simulink model "PV_Array_Application_R"  (Simulink 7.5)
settings: Solver=ode1  StartTime=0.0  StopTime=10.0  FixedStep=0.01  RelTol=1e-3
libraries: simulink x8, powerlib x4
settings Model: Creator=Leo216  LastModifiedBy=Leo216

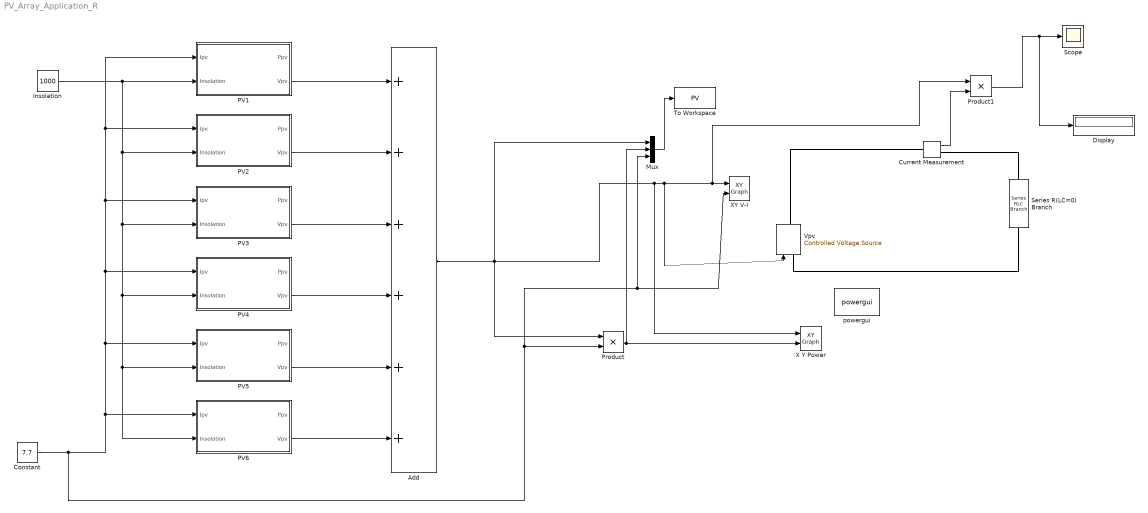
== system PV_Array_Application_R ==
  Add : Sum  Inputs=++++++  OutDataType=fixdt(1, 16)  OutScaling=2^-10
  Constant : Constant  Value=7.7  OutDataType=fixdt(1, 16)  OutScaling=2^0
  Current Measurement : powerlib/Measurements/Current Measurement  DialogController=POWERSYS.PowerSysDialog  SystemSampleTime=-1  PhasorSimulation=off  OutputType=Complex  PSBequivalent=0
  Display : Display
  Insolation : Constant  Value=1000  OutDataType=fixdt(1, 16)  OutScaling=2^0  SampleTime=-1
  Mux : Mux  Inputs=3
  PV1 : Subsystem  mask{Isc=8.4, Voc=39.6/63, Ir=7.7, Vr=31.9/63, Diode=on}
      mask prompts: Isc "Short-circuit current"; Voc "Open-Circuit Voltage"; Ir "Current at Pmax"; Vr "Voltage at Pmax"; Diode "By-pass diode"
      mask init:
      | Ns=round(Voc/0.61);
      | Vt=26e-3
      | G= Isc/1000;
      | Vmpc=Vr/Ns;
      | Vocc=Voc/Ns;
      | Rmpp=Vmpc/Ir;
      | 
      | Rp=100*Vocc/Isc;
      | Vdm=Vocc;
      | 
      | for i=1:10
      |     
      |    Idm=Isc-Ir-Vdm/Rp;
      |    Io=(Isc-Vocc/Rp)/(exp(Vocc/Vt)-1);
      |    Vdm=Vt*log(Idm/Io+1);
      |    Rs=(Vdm-Vmpc)/Ir;
      |    Rd=(Rmpp-Rs)*Rp/(Rp-Rmpp+Rs);
      |    Idm=Vt/Rd;
      |    Rp=Vdm/(Isc-Ir-Idm);
      |    
      | end
      mask Display: image(imread('pv.jpg'))
  PV2 : Subsystem  mask{Isc=8.4, Voc=39.6/63, Ir=7.7, Vr=31.9/63, Diode=on}
      mask prompts: Isc "Short-circuit current"; Voc "Open-Circuit Voltage"; Ir "Current at Pmax"; Vr "Voltage at Pmax"; Diode "By-pass diode"
      mask init: same as PV_Array_Application_R/PV1
      mask Display: image(imread('pv.jpg'))
  PV3 : Subsystem  mask{Isc=8.4, Voc=39.6/63, Ir=7.7, Vr=31.9/63, Diode=on}
      mask prompts: Isc "Short-circuit current"; Voc "Open-Circuit Voltage"; Ir "Current at Pmax"; Vr "Voltage at Pmax"; Diode "By-pass diode"
      mask init: same as PV_Array_Application_R/PV1
      mask Display: image(imread('pv.jpg'))
  PV4 : Subsystem  mask{Isc=8.4, Voc=39.6/63, Ir=7.7, Vr=31.9/63, Diode=on}
      mask prompts: Isc "Short-circuit current"; Voc "Open-Circuit Voltage"; Ir "Current at Pmax"; Vr "Voltage at Pmax"; Diode "By-pass diode"
      mask init: same as PV_Array_Application_R/PV1
      mask Display: image(imread('pv.jpg'))
  PV5 : Subsystem  mask{Isc=8.4, Voc=39.6/63, Ir=7.7, Vr=31.9/63, Diode=on}
      mask prompts: Isc "Short-circuit current"; Voc "Open-Circuit Voltage"; Ir "Current at Pmax"; Vr "Voltage at Pmax"; Diode "By-pass diode"
      mask init: same as PV_Array_Application_R/PV1
      mask Display: image(imread('pv.jpg'))
  PV6 : Subsystem  mask{Isc=8.4, Voc=39.6/63, Ir=7.7, Vr=31.9/63, Diode=on}
      mask prompts: Isc "Short-circuit current"; Voc "Open-Circuit Voltage"; Ir "Current at Pmax"; Vr "Voltage at Pmax"; Diode "By-pass diode"
      mask init: same as PV_Array_Application_R/PV1
      mask Display: image(imread('pv.jpg'))
  Product : Product  OutDataType=fixdt(1, 16)  OutScaling=2^0  RndMeth=Zero
  Product1 : Product  OutDataType=fixdt(1, 16)  OutScaling=2^0  RndMeth=Zero
  Scope : Scope
      settings: TimeRange=50
  Series R(LC=0) Branch : powerlib/Elements/Series RLC Branch  DialogController=POWERSYS.PowerSysDialog  PhysicalDomain=powersysdomain  SubClassName=unknown  LeftPortType=p1  RightPortType=p1  LConnTagsString=__new0  RConnTagsString=__new0  BranchType=R  Resistance=0.39  Inductance=1e-3  SetiL0=off  InitialCurrent=0  Capacitance=1e-6  Setx0=off  InitialVoltage=0  Measurements=None
  To Workspace : ToWorkspace  VariableName=PV  SampleTime=-1  SaveFormat=Structure
  Vpv : powerlib/Electrical Sources/Controlled Voltage Source  DialogController=POWERSYS.PowerSysDialog  SystemSampleTime=-1  Initialize=on  Source_Type=AC  Amplitude=0  Phase=0  Frequency=0  Measurements=None
  X Y Power : simulink/Sinks/XY Graph  SystemSampleTime=-1  xmin=0  xmax=10  ymin=0  ymax=10  st=-1
  XY V-I : simulink/Sinks/XY Graph  SystemSampleTime=-1  xmin=0  xmax=10  ymin=0  ymax=10  st=-1
  powergui : powerlib/powergui  Priority=1  SystemSampleTime=-1  SimulationMode=Continuous  SampleTime=50e-6  frequency=60  SPID=off  DisableSnubberDevices=off  DisableRonSwitches=off  DisableVfSwitches=off  SwTol=0  Interpol=off  frequencyindice=0  echomessages=off  HookPort=off  DisplayEquations=off  FunctionMessages=off  EnableUseOfTLC=off  x0status=blocks  RestoreLinks=warning  ResistiveCurrentMeasurement=off  Ylog=off  Xlog=on  ShowGrid=off  save=off  variable=ZData  ZoomFFT=off  StartTime=0.0  cycles=1  DisplayStyle=1  FreqAxis=off  MaxFrequency=1000  frequencyindicesteady=1  display=off  methode=off
  wires:
  PV1/2(Vpv) -> Add/1
  PV2/2(Vpv) -> Add/2
  PV3/2(Vpv) -> Add/3
  PV4/2(Vpv) -> Add/4
  PV5/2(Vpv) -> Add/5
  PV6/2(Vpv) -> Add/6
  Insolation/1 -> PV1/2(Insolation), PV5/2(Insolation), PV6/2(Insolation), PV4/2(Insolation), PV3/2(Insolation), PV2/2(Insolation)
  Constant/1 -> PV1/1(Ipv), PV2/1(Ipv), PV3/1(Ipv), PV4/1(Ipv), PV5/1(Ipv), PV6/1(Ipv), Product/2, XY V-I/2, Mux/3
  Product/1 -> X Y Power/2, Mux/2
  Mux/1 -> To Workspace/1
  Add/1 -> Mux/1, X Y Power/1, Vpv/1, XY V-I/1, Product1/1, Product/1
  Current Measurement/1 -> Product1/2
  Product1/1 -> Scope/1, Display/1
  connections:
  Vpv/LConn1 -- Series R(LC=0) Branch/RConn1
  Vpv/RConn1 -- Current Measurement/LConn1
  Current Measurement/RConn1 -- Series R(LC=0) Branch/LConn1

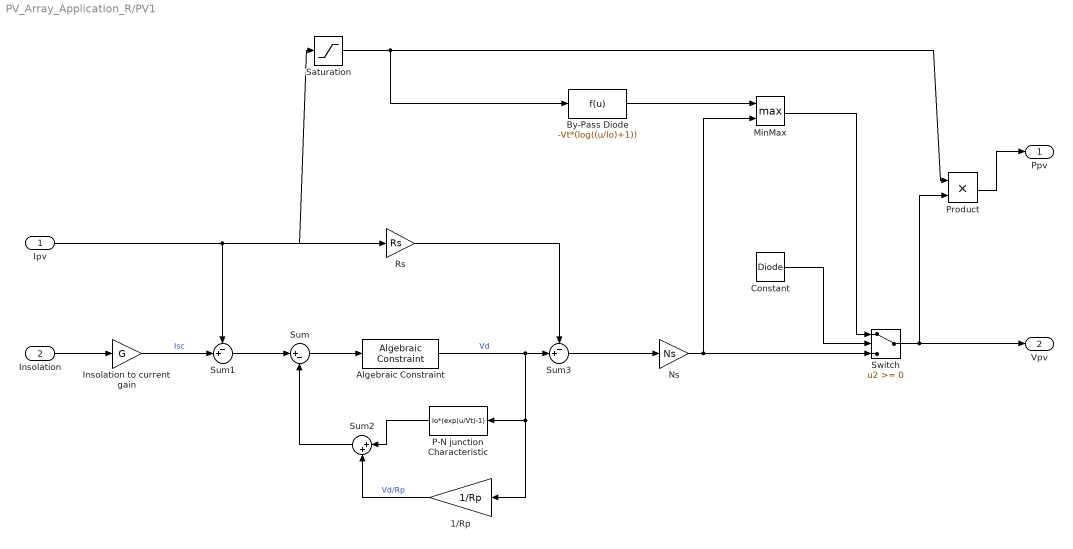
== system PV_Array_Application_R/PV1 ==
  Ipv : Inport  OutDataType=fixdt(1, 16)  OutScaling=2^0
  Insolation : Inport  Port=2  OutDataType=fixdt(1, 16)  OutScaling=2^0
  1/Rp : Gain  Gain=1/Rp  ParameterDataType=fixdt(1, 16)  ParameterScaling=2^0  OutDataType=fixdt(1, 16)  OutScaling=2^0
  Algebraic Constraint : simulink/Math Operations/Algebraic Constraint  SystemSampleTime=-1  z0=0.5
  By-Pass Diode : Fcn  Expr=-Vt*(log((u/Io)+1))
  Constant : Constant  Value=Diode  OutDataType=fixdt(1, 16)  OutScaling=2^0  SampleTime=-1
  Insolation to current gain : Gain  Gain=G  ParameterDataType=fixdt(1, 16)  ParameterScaling=2^0  OutDataType=fixdt(1, 16)  OutScaling=2^0
  MinMax : MinMax  Function=max  Inputs=2  OutDataType=fixdt(1, 16)  OutScaling=2^0
  Ns : Gain  Gain=Ns  ParameterDataType=fixdt(1, 16)  ParameterScaling=2^0  OutDataType=fixdt(1, 16)  OutScaling=2^0
  P-N junction Characteristic : Fcn  Expr=Io*(exp(u/Vt)-1)
  Product : Product  OutDataType=fixdt(1, 16)  OutScaling=2^0  RndMeth=Zero
  Rs : Gain  Gain=Rs  ParameterDataType=fixdt(1, 16)  ParameterScaling=2^0  OutDataType=fixdt(1, 16)  OutScaling=2^0
  Saturation : Saturate  OutDataType=fixdt(1, 16)  OutScaling=2^0
  Sum : Sum  Inputs=|+-  OutDataType=fixdt(1, 16)  OutScaling=2^0
  Sum1 : Sum  Inputs=-+|  OutDataType=fixdt(1, 16)  OutScaling=2^0
  Sum2 : Sum  Inputs=|++  OutDataType=fixdt(1, 16)  OutScaling=2^0
  Sum3 : Sum  Inputs=-+|  OutDataType=fixdt(1, 16)  OutScaling=2^0
  Switch : Switch  OutDataType=fixdt(1, 16)  OutScaling=2^0
  Ppv : Outport  OutDataType=fixdt(1, 16)  OutScaling=2^0
  Vpv : Outport  Port=2  OutDataType=fixdt(1, 16)  OutScaling=2^0
  wires:
  Insolation/1 -> Insolation to current gain/1
  Product/1 -> Ppv/1
  By-Pass Diode/1 -> MinMax/1
  P-N junction Characteristic/1 -> Sum2/1
  Saturation/1 -> Product/1, By-Pass Diode/1
  Switch/1 -> Product/2, Vpv/1
  MinMax/1 -> Switch/1
  Constant/1 -> Switch/2
  Ns/1 -> Switch/3, MinMax/2
  Sum3/1 -> Ns/1
  Rs/1 -> Sum3/1
  Algebraic Constraint/1 -> Sum3/2, 1/Rp/1, P-N junction Characteristic/1  "Vd"
  1/Rp/1 -> Sum2/2  "Vd/Rp"
  Sum2/1 -> Sum/2
  Sum/1 -> Algebraic Constraint/1
  Sum1/1 -> Sum/1
  Insolation to current gain/1 -> Sum1/2  "Isc"
  Ipv/1 -> Sum1/1, Rs/1, Saturation/1

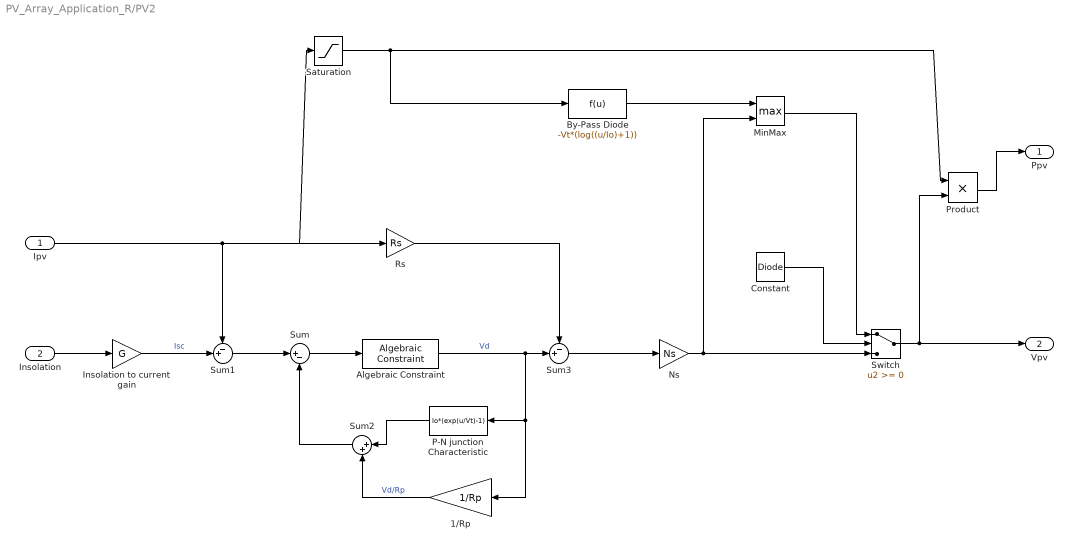
== system PV_Array_Application_R/PV2 ==
  Ipv : Inport  OutDataType=fixdt(1, 16)  OutScaling=2^0
  Insolation : Inport  Port=2  OutDataType=fixdt(1, 16)  OutScaling=2^0
  1/Rp : Gain  Gain=1/Rp  ParameterDataType=fixdt(1, 16)  ParameterScaling=2^0  OutDataType=fixdt(1, 16)  OutScaling=2^0
  Algebraic Constraint : simulink/Math Operations/Algebraic Constraint  SystemSampleTime=-1  z0=0
  By-Pass Diode : Fcn  Expr=-Vt*(log((u/Io)+1))
  Constant : Constant  Value=Diode  OutDataType=fixdt(1, 16)  OutScaling=2^0  SampleTime=-1
  Insolation to current gain : Gain  Gain=G  ParameterDataType=fixdt(1, 16)  ParameterScaling=2^0  OutDataType=fixdt(1, 16)  OutScaling=2^0
  MinMax : MinMax  Function=max  Inputs=2  OutDataType=fixdt(1, 16)  OutScaling=2^0
  Ns : Gain  Gain=Ns  ParameterDataType=fixdt(1, 16)  ParameterScaling=2^0  OutDataType=fixdt(1, 16)  OutScaling=2^0
  P-N junction Characteristic : Fcn  Expr=Io*(exp(u/Vt)-1)
  Product : Product  OutDataType=fixdt(1, 16)  OutScaling=2^0  RndMeth=Zero
  Rs : Gain  Gain=Rs  ParameterDataType=fixdt(1, 16)  ParameterScaling=2^0  OutDataType=fixdt(1, 16)  OutScaling=2^0
  Saturation : Saturate  OutDataType=fixdt(1, 16)  OutScaling=2^0
  Sum : Sum  Inputs=|+-  OutDataType=fixdt(1, 16)  OutScaling=2^0
  Sum1 : Sum  Inputs=-+|  OutDataType=fixdt(1, 16)  OutScaling=2^0
  Sum2 : Sum  Inputs=|++  OutDataType=fixdt(1, 16)  OutScaling=2^0
  Sum3 : Sum  Inputs=-+|  OutDataType=fixdt(1, 16)  OutScaling=2^0
  Switch : Switch  OutDataType=fixdt(1, 16)  OutScaling=2^0
  Ppv : Outport  OutDataType=fixdt(1, 16)  OutScaling=2^0
  Vpv : Outport  Port=2  OutDataType=fixdt(1, 16)  OutScaling=2^0
  wires:
  Insolation/1 -> Insolation to current gain/1
  Product/1 -> Ppv/1
  By-Pass Diode/1 -> MinMax/1
  P-N junction Characteristic/1 -> Sum2/1
  Saturation/1 -> Product/1, By-Pass Diode/1
  Switch/1 -> Product/2, Vpv/1
  MinMax/1 -> Switch/1
  Constant/1 -> Switch/2
  Ns/1 -> Switch/3, MinMax/2
  Sum3/1 -> Ns/1
  Rs/1 -> Sum3/1
  Algebraic Constraint/1 -> Sum3/2, 1/Rp/1, P-N junction Characteristic/1  "Vd"
  1/Rp/1 -> Sum2/2  "Vd/Rp"
  Sum2/1 -> Sum/2
  Sum/1 -> Algebraic Constraint/1
  Sum1/1 -> Sum/1
  Insolation to current gain/1 -> Sum1/2  "Isc"
  Ipv/1 -> Sum1/1, Rs/1, Saturation/1

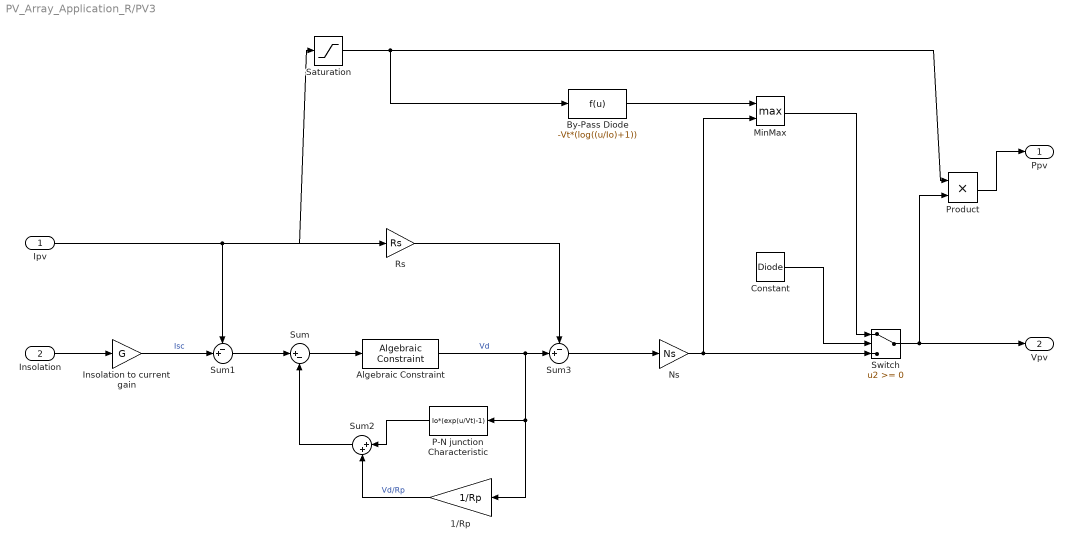
== system PV_Array_Application_R/PV3 ==
  Ipv : Inport  OutDataType=fixdt(1, 16)  OutScaling=2^0
  Insolation : Inport  Port=2  OutDataType=fixdt(1, 16)  OutScaling=2^0
  1/Rp : Gain  Gain=1/Rp  ParameterDataType=fixdt(1, 16)  ParameterScaling=2^0  OutDataType=fixdt(1, 16)  OutScaling=2^0
  Algebraic Constraint : simulink/Math Operations/Algebraic Constraint  SystemSampleTime=-1  z0=0
  By-Pass Diode : Fcn  Expr=-Vt*(log((u/Io)+1))
  Constant : Constant  Value=Diode  OutDataType=fixdt(1, 16)  OutScaling=2^0  SampleTime=-1
  Insolation to current gain : Gain  Gain=G  ParameterDataType=fixdt(1, 16)  ParameterScaling=2^0  OutDataType=fixdt(1, 16)  OutScaling=2^0
  MinMax : MinMax  Function=max  Inputs=2  OutDataType=fixdt(1, 16)  OutScaling=2^0
  Ns : Gain  Gain=Ns  ParameterDataType=fixdt(1, 16)  ParameterScaling=2^0  OutDataType=fixdt(1, 16)  OutScaling=2^0
  P-N junction Characteristic : Fcn  Expr=Io*(exp(u/Vt)-1)
  Product : Product  OutDataType=fixdt(1, 16)  OutScaling=2^0  RndMeth=Zero
  Rs : Gain  Gain=Rs  ParameterDataType=fixdt(1, 16)  ParameterScaling=2^0  OutDataType=fixdt(1, 16)  OutScaling=2^0
  Saturation : Saturate  OutDataType=fixdt(1, 16)  OutScaling=2^0
  Sum : Sum  Inputs=|+-  OutDataType=fixdt(1, 16)  OutScaling=2^0
  Sum1 : Sum  Inputs=-+|  OutDataType=fixdt(1, 16)  OutScaling=2^0
  Sum2 : Sum  Inputs=|++  OutDataType=fixdt(1, 16)  OutScaling=2^0
  Sum3 : Sum  Inputs=-+|  OutDataType=fixdt(1, 16)  OutScaling=2^0
  Switch : Switch  OutDataType=fixdt(1, 16)  OutScaling=2^0
  Ppv : Outport  OutDataType=fixdt(1, 16)  OutScaling=2^0
  Vpv : Outport  Port=2  OutDataType=fixdt(1, 16)  OutScaling=2^0
  wires:
  Insolation/1 -> Insolation to current gain/1
  Product/1 -> Ppv/1
  By-Pass Diode/1 -> MinMax/1
  P-N junction Characteristic/1 -> Sum2/1
  Saturation/1 -> Product/1, By-Pass Diode/1
  Switch/1 -> Product/2, Vpv/1
  MinMax/1 -> Switch/1
  Constant/1 -> Switch/2
  Ns/1 -> Switch/3, MinMax/2
  Sum3/1 -> Ns/1
  Rs/1 -> Sum3/1
  Algebraic Constraint/1 -> Sum3/2, 1/Rp/1, P-N junction Characteristic/1  "Vd"
  1/Rp/1 -> Sum2/2  "Vd/Rp"
  Sum2/1 -> Sum/2
  Sum/1 -> Algebraic Constraint/1
  Sum1/1 -> Sum/1
  Insolation to current gain/1 -> Sum1/2  "Isc"
  Ipv/1 -> Sum1/1, Rs/1, Saturation/1

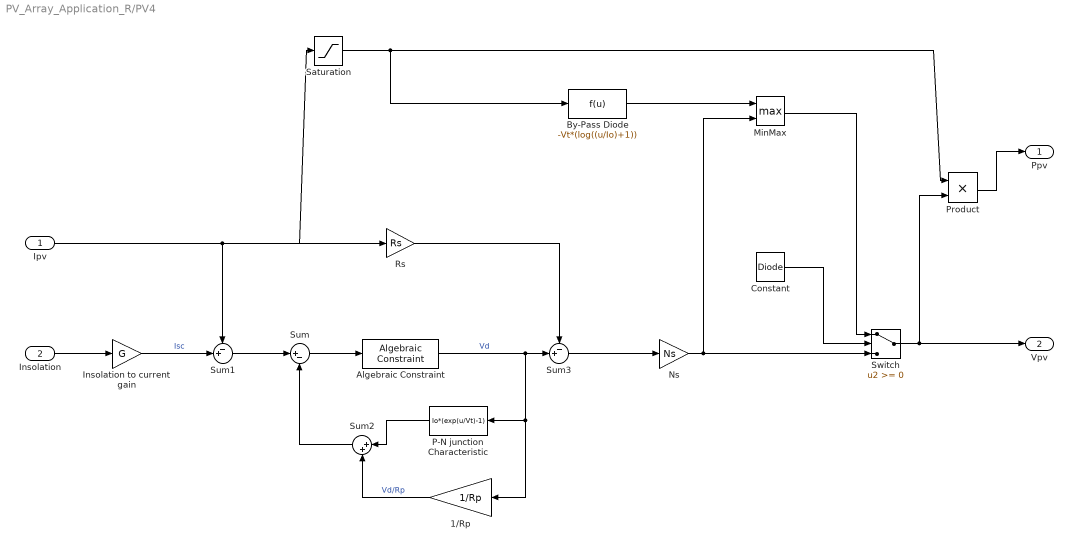
== system PV_Array_Application_R/PV4 ==
  Ipv : Inport  OutDataType=fixdt(1, 16)  OutScaling=2^0
  Insolation : Inport  Port=2  OutDataType=fixdt(1, 16)  OutScaling=2^0
  1/Rp : Gain  Gain=1/Rp  ParameterDataType=fixdt(1, 16)  ParameterScaling=2^0  OutDataType=fixdt(1, 16)  OutScaling=2^0
  Algebraic Constraint : simulink/Math Operations/Algebraic Constraint  SystemSampleTime=-1  z0=0
  By-Pass Diode : Fcn  Expr=-Vt*(log((u/Io)+1))
  Constant : Constant  Value=Diode  OutDataType=fixdt(1, 16)  OutScaling=2^0
  Insolation to current gain : Gain  Gain=G  ParameterDataType=fixdt(1, 16)  ParameterScaling=2^0  OutDataType=fixdt(1, 16)  OutScaling=2^0
  MinMax : MinMax  Function=max  Inputs=2  OutDataType=fixdt(1, 16)  OutScaling=2^0
  Ns : Gain  Gain=Ns  ParameterDataType=fixdt(1, 16)  ParameterScaling=2^0  OutDataType=fixdt(1, 16)  OutScaling=2^0
  P-N junction Characteristic : Fcn  Expr=Io*(exp(u/Vt)-1)
  Product : Product  OutDataType=fixdt(1, 16)  OutScaling=2^0  RndMeth=Zero
  Rs : Gain  Gain=Rs  ParameterDataType=fixdt(1, 16)  ParameterScaling=2^0  OutDataType=fixdt(1, 16)  OutScaling=2^0
  Saturation : Saturate  OutDataType=fixdt(1, 16)  OutScaling=2^0
  Sum : Sum  Inputs=|+-  OutDataType=fixdt(1, 16)  OutScaling=2^0
  Sum1 : Sum  Inputs=-+|  OutDataType=fixdt(1, 16)  OutScaling=2^0
  Sum2 : Sum  Inputs=|++  OutDataType=fixdt(1, 16)  OutScaling=2^0
  Sum3 : Sum  Inputs=-+|  OutDataType=fixdt(1, 16)  OutScaling=2^0
  Switch : Switch  OutDataType=fixdt(1, 16)  OutScaling=2^0
  Ppv : Outport  OutDataType=fixdt(1, 16)  OutScaling=2^0
  Vpv : Outport  Port=2  OutDataType=fixdt(1, 16)  OutScaling=2^0
  wires:
  Insolation/1 -> Insolation to current gain/1
  Product/1 -> Ppv/1
  By-Pass Diode/1 -> MinMax/1
  P-N junction Characteristic/1 -> Sum2/1
  Saturation/1 -> Product/1, By-Pass Diode/1
  Switch/1 -> Product/2, Vpv/1
  MinMax/1 -> Switch/1
  Constant/1 -> Switch/2
  Ns/1 -> Switch/3, MinMax/2
  Sum3/1 -> Ns/1
  Rs/1 -> Sum3/1
  Algebraic Constraint/1 -> Sum3/2, 1/Rp/1, P-N junction Characteristic/1  "Vd"
  1/Rp/1 -> Sum2/2  "Vd/Rp"
  Sum2/1 -> Sum/2
  Sum/1 -> Algebraic Constraint/1
  Sum1/1 -> Sum/1
  Insolation to current gain/1 -> Sum1/2  "Isc"
  Ipv/1 -> Sum1/1, Rs/1, Saturation/1

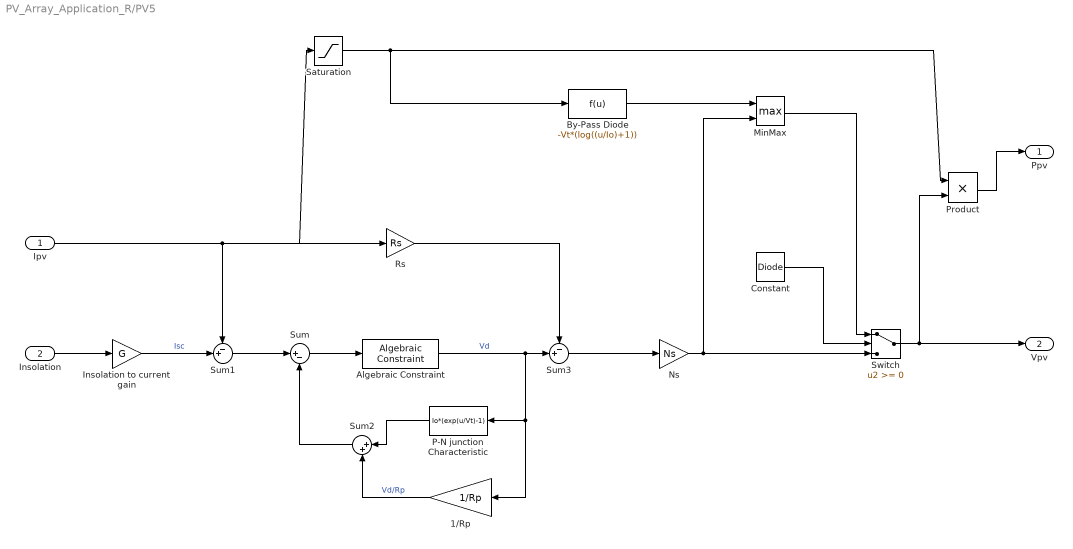
== system PV_Array_Application_R/PV5 ==
  Ipv : Inport  OutDataType=fixdt(1, 16)  OutScaling=2^0
  Insolation : Inport  Port=2  OutDataType=fixdt(1, 16)  OutScaling=2^0
  1/Rp : Gain  Gain=1/Rp  ParameterDataType=fixdt(1, 16)  ParameterScaling=2^0  OutDataType=fixdt(1, 16)  OutScaling=2^0
  Algebraic Constraint : simulink/Math Operations/Algebraic Constraint  SystemSampleTime=-1  z0=0
  By-Pass Diode : Fcn  Expr=-Vt*(log((u/Io)+1))
  Constant : Constant  Value=Diode  OutDataType=fixdt(1, 16)  OutScaling=2^0
  Insolation to current gain : Gain  Gain=G  ParameterDataType=fixdt(1, 16)  ParameterScaling=2^0  OutDataType=fixdt(1, 16)  OutScaling=2^0
  MinMax : MinMax  Function=max  Inputs=2  OutDataType=fixdt(1, 16)  OutScaling=2^0
  Ns : Gain  Gain=Ns  ParameterDataType=fixdt(1, 16)  ParameterScaling=2^0  OutDataType=fixdt(1, 16)  OutScaling=2^0
  P-N junction Characteristic : Fcn  Expr=Io*(exp(u/Vt)-1)
  Product : Product  OutDataType=fixdt(1, 16)  OutScaling=2^0  RndMeth=Zero
  Rs : Gain  Gain=Rs  ParameterDataType=fixdt(1, 16)  ParameterScaling=2^0  OutDataType=fixdt(1, 16)  OutScaling=2^0
  Saturation : Saturate  OutDataType=fixdt(1, 16)  OutScaling=2^0
  Sum : Sum  Inputs=|+-  OutDataType=fixdt(1, 16)  OutScaling=2^0
  Sum1 : Sum  Inputs=-+|  OutDataType=fixdt(1, 16)  OutScaling=2^0
  Sum2 : Sum  Inputs=|++  OutDataType=fixdt(1, 16)  OutScaling=2^0
  Sum3 : Sum  Inputs=-+|  OutDataType=fixdt(1, 16)  OutScaling=2^0
  Switch : Switch  OutDataType=fixdt(1, 16)  OutScaling=2^0
  Ppv : Outport  OutDataType=fixdt(1, 16)  OutScaling=2^0
  Vpv : Outport  Port=2  OutDataType=fixdt(1, 16)  OutScaling=2^0
  wires:
  Insolation/1 -> Insolation to current gain/1
  Product/1 -> Ppv/1
  By-Pass Diode/1 -> MinMax/1
  P-N junction Characteristic/1 -> Sum2/1
  Saturation/1 -> Product/1, By-Pass Diode/1
  Switch/1 -> Product/2, Vpv/1
  MinMax/1 -> Switch/1
  Constant/1 -> Switch/2
  Ns/1 -> Switch/3, MinMax/2
  Sum3/1 -> Ns/1
  Rs/1 -> Sum3/1
  Algebraic Constraint/1 -> Sum3/2, 1/Rp/1, P-N junction Characteristic/1  "Vd"
  1/Rp/1 -> Sum2/2  "Vd/Rp"
  Sum2/1 -> Sum/2
  Sum/1 -> Algebraic Constraint/1
  Sum1/1 -> Sum/1
  Insolation to current gain/1 -> Sum1/2  "Isc"
  Ipv/1 -> Sum1/1, Rs/1, Saturation/1

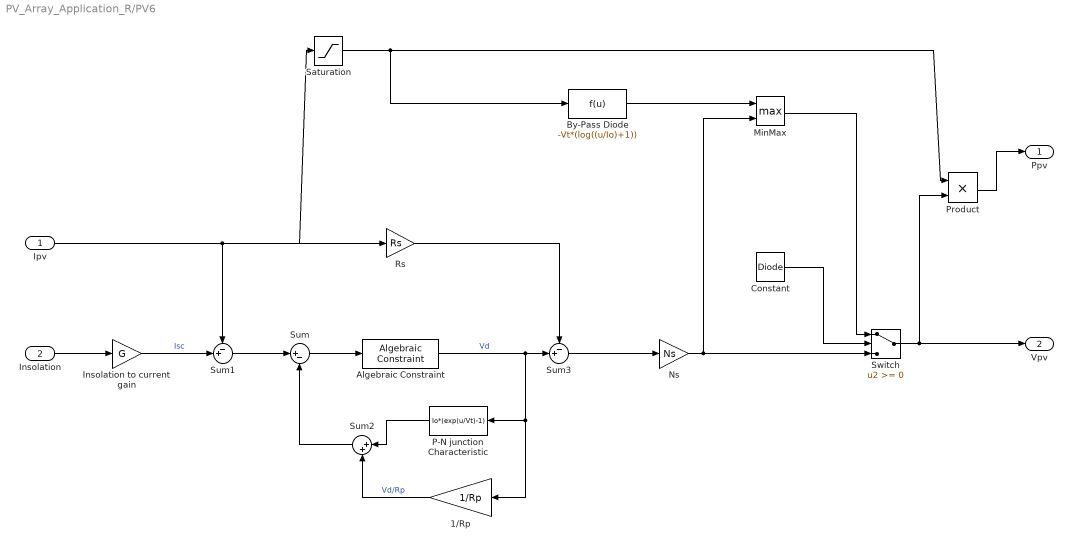
== system PV_Array_Application_R/PV6 ==
  Ipv : Inport  OutDataType=fixdt(1, 16)  OutScaling=2^0
  Insolation : Inport  Port=2  OutDataType=fixdt(1, 16)  OutScaling=2^0
  1/Rp : Gain  Gain=1/Rp  ParameterDataType=fixdt(1, 16)  ParameterScaling=2^0  OutDataType=fixdt(1, 16)  OutScaling=2^0
  Algebraic Constraint : simulink/Math Operations/Algebraic Constraint  SystemSampleTime=-1  z0=0
  By-Pass Diode : Fcn  Expr=-Vt*(log((u/Io)+1))
  Constant : Constant  Value=Diode  OutDataType=fixdt(1, 16)  OutScaling=2^0
  Insolation to current gain : Gain  Gain=G  ParameterDataType=fixdt(1, 16)  ParameterScaling=2^0  OutDataType=fixdt(1, 16)  OutScaling=2^0
  MinMax : MinMax  Function=max  Inputs=2  OutDataType=fixdt(1, 16)  OutScaling=2^0
  Ns : Gain  Gain=Ns  ParameterDataType=fixdt(1, 16)  ParameterScaling=2^0  OutDataType=fixdt(1, 16)  OutScaling=2^0
  P-N junction Characteristic : Fcn  Expr=Io*(exp(u/Vt)-1)
  Product : Product  OutDataType=fixdt(1, 16)  OutScaling=2^0  RndMeth=Zero
  Rs : Gain  Gain=Rs  ParameterDataType=fixdt(1, 16)  ParameterScaling=2^0  OutDataType=fixdt(1, 16)  OutScaling=2^0
  Saturation : Saturate  OutDataType=fixdt(1, 16)  OutScaling=2^0
  Sum : Sum  Inputs=|+-  OutDataType=fixdt(1, 16)  OutScaling=2^0
  Sum1 : Sum  Inputs=-+|  OutDataType=fixdt(1, 16)  OutScaling=2^0
  Sum2 : Sum  Inputs=|++  OutDataType=fixdt(1, 16)  OutScaling=2^0
  Sum3 : Sum  Inputs=-+|  OutDataType=fixdt(1, 16)  OutScaling=2^0
  Switch : Switch  OutDataType=fixdt(1, 16)  OutScaling=2^0
  Ppv : Outport  OutDataType=fixdt(1, 16)  OutScaling=2^0
  Vpv : Outport  Port=2  OutDataType=fixdt(1, 16)  OutScaling=2^0
  wires:
  Insolation/1 -> Insolation to current gain/1
  Product/1 -> Ppv/1
  By-Pass Diode/1 -> MinMax/1
  P-N junction Characteristic/1 -> Sum2/1
  Saturation/1 -> Product/1, By-Pass Diode/1
  Switch/1 -> Product/2, Vpv/1
  MinMax/1 -> Switch/1
  Constant/1 -> Switch/2
  Ns/1 -> Switch/3, MinMax/2
  Sum3/1 -> Ns/1
  Rs/1 -> Sum3/1
  Algebraic Constraint/1 -> Sum3/2, 1/Rp/1, P-N junction Characteristic/1  "Vd"
  1/Rp/1 -> Sum2/2  "Vd/Rp"
  Sum2/1 -> Sum/2
  Sum/1 -> Algebraic Constraint/1
  Sum1/1 -> Sum/1
  Insolation to current gain/1 -> Sum1/2  "Isc"
  Ipv/1 -> Sum1/1, Rs/1, Saturation/1
